simulink model "FINAL_SIMULATION"  (R2017a)
settings: Solver=FixedStepDiscrete  StartTime=0.0  StopTime=1  FixedStep=1e-6  RelTol=1e-3
libraries: powerlib x18, simulink x2, powerlib_meascontrol x2
settings Model: Creator=M. Mahinur Rahman  LastModifiedBy=Junaed

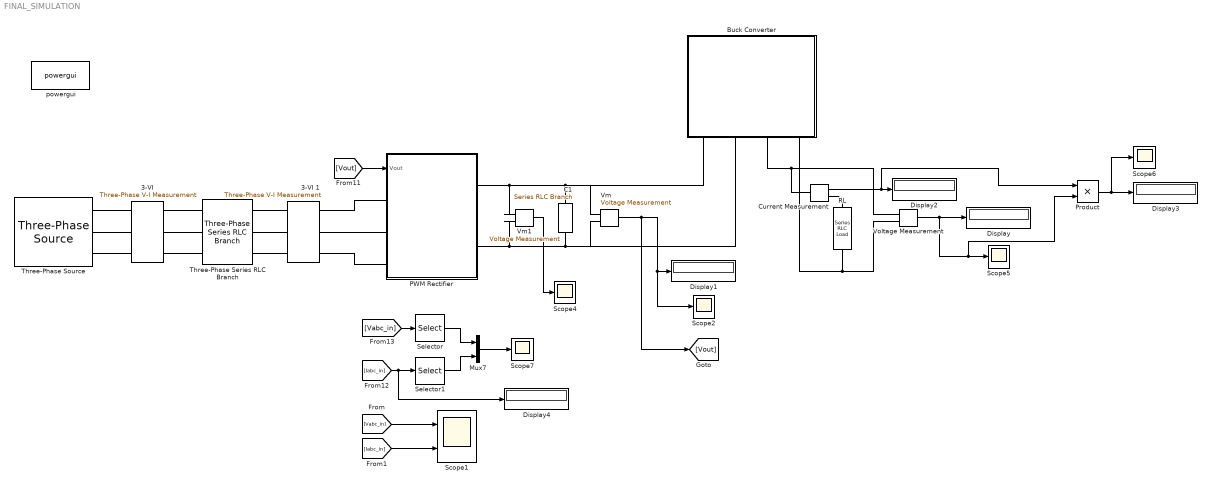
== system FINAL_SIMULATION ==
  " RL" : powerlib/Elements/Series RLC Load  LConnTagsString=a  RConnTagsString=__new0  NominalVoltage=87  NominalFrequency=50  ActivePower=2e3  InductivePower=0  CapacitivePower=0  Setx0=off  InitialVoltage=0  SetiL0=off  InitialCurrent=0  Measurements=None  LoadType=constant Z
  "3-VI " : powerlib/Measurements/Three-Phase V-I Measurement  VoltageMeasurement=phase-to-ground  SetLabelV=on  LabelV=Vabc_in  Vpu=off  VpuLL=off  CurrentMeasurement=yes  SetLabelI=on  LabelI=Iabc_in  Ipu=off  Pbase=100e6  Vbase=500e3  OutputType=Complex  PhasorSimulation=off  PSBequivalent=0
  3-VI 1 : powerlib/Measurements/Three-Phase V-I Measurement  VoltageMeasurement=phase-to-ground  SetLabelV=on  LabelV=Vabc_sw  Vpu=off  VpuLL=off  CurrentMeasurement=yes  SetLabelI=on  LabelI=Iabc_sw  Ipu=off  Pbase=100e6  Vbase=500e3  OutputType=Complex  PhasorSimulation=off  PSBequivalent=0
  Buck Converter : Subsystem
  C1 : powerlib/Elements/Series RLC Branch  LConnTagsString=__new0  RConnTagsString=__new0  BranchType=C  Resistance=1  Inductance=1e-3  SetiL0=off  InitialCurrent=0  Capacitance=1000e-6  Setx0=off  InitialVoltage=0  Measurements=None
  Current Measurement : powerlib/Measurements/Current Measurement  PhasorSimulation=off  OutputType=Complex  PSBequivalent=0
  Display{,1..4} (5 alike) : Display
  Mux7 : Mux  Inputs=2
  "PWM Rectifier " : Subsystem
  Product : Product
  Scope1 : Scope  NumInputPorts=2
  Scope{2,4..7} (5 alike) : Scope
  Selector : Selector  InputPortWidth=3  IndexOptions=Index vector (dialog)  Indices=[1]  OutputSizes=1
  Selector1 : Selector  InputPortWidth=3  IndexOptions=Index vector (dialog)  Indices=[1]  OutputSizes=1
  Three-Phase Series RLC Branch : powerlib/Elements/Three-Phase Series RLC Branch  LConnTagsString=A|B|C  RConnTagsString=A|B|C  BranchType=RL  Resistance=1  Inductance=5e-3  Capacitance=1e-6  Measurements=None
  Three-Phase Source : powerlib/Electrical Sources/Three-Phase Source  InternalConnection=Yg  VoltagePhases=off  Voltage=400  PhaseAngle=0  Voltage_phases=[25e3 25e3 25e3]/sqrt(3)  PhaseAngles_phases=[0 -120 +120]  Frequency=50  NonIdealSource=off  SpecifyImpedance=off  Resistance=0.8929  Inductance=16.58e-3  ShortCircuitLevel=100e6  BaseVoltage=25e3  XRratio=7  BusType=swing  Pref=10e3  Qref=0  Prefabc=[10e3, 10e3, 10e3]  Qrefabc=[0, 0, 0]  Qmin=-inf  Qmax=inf
  Vm : powerlib/Measurements/Voltage Measurement  PhasorSimulation=off  OutputType=Complex  PSBequivalent=0
  Vm1 : powerlib/Measurements/Voltage Measurement  PhasorSimulation=off  OutputType=Complex  PSBequivalent=0
  Voltage Measurement : powerlib/Measurements/Voltage Measurement  PhasorSimulation=off  OutputType=Complex  PSBequivalent=0
  powergui : powerlib/powergui  Priority=1  SimulationMode=Discrete  SampleTime=1e-6  frequency=60  Iterations=50  frequencyindice=50  Pbase=100e6  ErrMax=1e-4  UnitsV=kV  UnitsW=MW  buscounter=0  FunctionMessages=off  echomessages=off  EnableUseOfTLC=off  CurrentSourceSwitches=off  DisableSnubberDevices=off  DisableRonSwitches=off  DisableVfSwitches=off  DisplayEquations=off  SolverType=Tustin/Backward Euler (TBE)  Interpol=off  ExternalGateDelay=off  methode=off  Ts=100  x0status=blocks  SPID=off  SwTol=0  HookPort=off  RestoreLinks=warning  ResistiveCurrentMeasurement=off  Frange=[0:2:500]  Ylog=off  Xlog=on  ShowGrid=off  save=off  variable=ZData  structure=0  ZoomFFT=off  StartTime=0.0  cycles=1  DisplayStyle=1  fundamental=60  FreqAxis=off  MaxFrequency=1000  frequencyindicesteady=1  RmsSteady=1  display=off
  wires:
  [Iabc_in] -> Scope1/2
  [Vabc_in] -> Scope1/1
  Vm1/1 -> Scope4/1
  [Vabc_in] -> Selector/1
  [Iabc_in] -> Display4/1, Selector1/1
  Selector/1 -> Mux7/1
  Selector1/1 -> Mux7/2
  Mux7/1 -> Scope7/1
  Voltage Measurement/1 -> Display/1, Product/2, Scope5/1
  [Vout] -> "PWM Rectifier "/1(Vout)
  Vm/1 -> Scope2/1, Display1/1, [Vout]
  Current Measurement/1 -> Product/1, Display2/1
  Product/1 -> Scope6/1, Display3/1
  connections:
  C1/LConn1 -- Vm/LConn1 -- Buck Converter/LConn1 -- Vm1/LConn1 -- "PWM Rectifier "/RConn1
  C1/RConn1 -- Vm/LConn2 -- Buck Converter/LConn2 -- Vm1/LConn2 -- "PWM Rectifier "/RConn2
  "3-VI "/LConn1 -- Three-Phase Source/RConn1
  Three-Phase Source/RConn2 -- "3-VI "/LConn2
  Three-Phase Source/RConn3 -- "3-VI "/LConn3
  "3-VI "/RConn1 -- Three-Phase Series RLC Branch/LConn1
  "3-VI "/RConn2 -- Three-Phase Series RLC Branch/LConn2
  "3-VI "/RConn3 -- Three-Phase Series RLC Branch/LConn3
  3-VI 1/LConn3 -- Three-Phase Series RLC Branch/RConn3
  3-VI 1/LConn2 -- Three-Phase Series RLC Branch/RConn2
  3-VI 1/LConn1 -- Three-Phase Series RLC Branch/RConn1
  3-VI 1/RConn1 -- "PWM Rectifier "/LConn1
  3-VI 1/RConn2 -- "PWM Rectifier "/LConn2
  3-VI 1/RConn3 -- "PWM Rectifier "/LConn3
  Voltage Measurement/LConn1 -- Current Measurement/LConn1 -- Buck Converter/LConn3
  " RL"/RConn1 -- Voltage Measurement/LConn2 -- Buck Converter/LConn4
  Current Measurement/RConn1 -- " RL"/LConn1

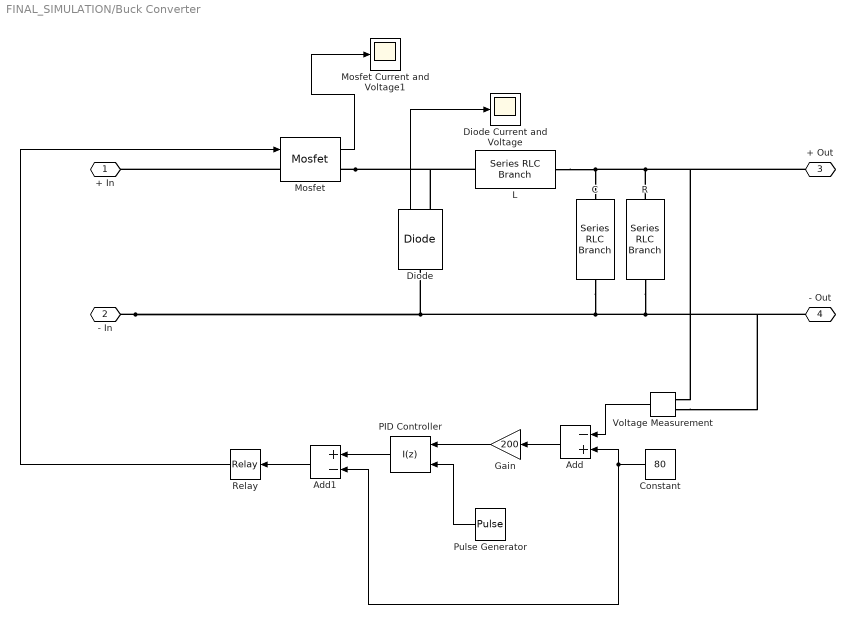
== system FINAL_SIMULATION/Buck Converter ==
  Add : Sum  Inputs=-+
  Add1 : Sum  Inputs=+-
  C : powerlib/Elements/Series RLC Branch  LConnTagsString=__new0  RConnTagsString=__new0  BranchType=C  Resistance=1  Inductance=1e-3  SetiL0=off  InitialCurrent=0  Capacitance=2.5e-5  Setx0=off  InitialVoltage=0  Measurements=None
  Constant : Constant  Value=80
  Diode : powerlib/Power Electronics/Diode  Ron=0.001  Lon=0  Vf=0.8  IC=0  UseSnubber=0  Rs=500  Cs=250e-9  Measurements=on
  Diode Current and Voltage : Scope
  Gain : Gain  Gain=200
  L : powerlib/Elements/Series RLC Branch  LConnTagsString=__new0  RConnTagsString=__new0  BranchType=L  Resistance=1  Inductance=0.34182  SetiL0=off  InitialCurrent=0  Capacitance=1e-6  Setx0=off  InitialVoltage=0  Measurements=None
  Mosfet : powerlib/Power Electronics/Mosfet  Ron=0.1  Lon=0  Rd=0.01  Vfd=0  IC=0  Rs=1e5  Cs=inf  Measurements=on
  Mosfet Current and Voltage1 : Scope
  PID Controller : simulink/Continuous/PID Controller  Controller=I  TimeDomain=Discrete-time  SampleTime=-1  IntegratorMethod=Forward Euler  FilterMethod=Forward Euler  Form=Parallel  UseFilter=on  ControllerParametersSource=internal  P=.001  I=40000  D=0  N=100  InitialConditionSource=internal  InitialConditionForIntegrator=0  InitialConditionForFilter=0  ExternalReset=falling  LimitOutput=off  UpperSaturationLimit=inf  LowerSaturationLimit=-inf  LinearizeAsGain=on  AntiWindupMode=none  Kb=1  TrackingMode=off  Kt=1  PParamMin=[]  PParamMax=[]  IParamMin=[]  IParamMax=[]  DParamMin=[]  DParamMax=[]  NParamMin=[]  NParamMax=[]  KbParamMin=[]  KbParamMax=[]  KtParamMin=[]  KtParamMax=[]  POutMin=[]  POutMax=[]  IOutMin=[]  IOutMax=[]  DOutMin=[]  DOutMax=[]  NOutMin=[]  NOutMax=[]  KbOutMin=[]  KbOutMax=[]  KtOutMin=[]  KtOutMax=[]  IntegratorOutMin=[]  IntegratorOutMax=[]  FilterOutMin=[]  FilterOutMax=[]  SumOutMin=[]  SumOutMax=[]  SumI1OutMin=[]  SumI1OutMax=[]  SumI2OutMin=[]  SumI2OutMax=[]  SumI3OutMin=[]  SumI3OutMax=[]  SumDOutMin=[]  SumDOutMax=[]  SaturationOutMin=[]  SaturationOutMax=[]  IntegratorContinuousStateAttributes=''  IntegratorStateMustResolveToSignalObject=off  IntegratorRTWStateStorageClass=Auto  FilterContinuousStateAttributes=''  FilterStateMustResolveToSignalObject=off  FilterRTWStateStorageClass=Auto  DifferentiatorICPrevScaledInput=0  DifferentiatorOutMin=[]  DifferentiatorOutMax=[]  InitialConditionSetting=State (most efficient)
  Pulse Generator : DiscretePulseGenerator  PulseType=Time based  Period=1/10000  PulseWidth=20
  R : powerlib/Elements/Series RLC Branch  LConnTagsString=__new0  RConnTagsString=__new0  BranchType=R  Resistance=20  Inductance=1e-3  SetiL0=off  InitialCurrent=0  Capacitance=1e-6  Setx0=off  InitialVoltage=0  Measurements=None
  Relay : Relay
  Voltage Measurement : powerlib/Measurements/Voltage Measurement  PhasorSimulation=off  OutputType=Complex  PSBequivalent=0
  + In : PMIOPort  Port=1  Side=Left
  - In : PMIOPort  Port=2  Side=Left
  + Out : PMIOPort  Port=3  Side=Left
  - Out : PMIOPort  Port=4  Side=Left
  wires:
  Diode/1 -> Diode Current and Voltage/1
  Mosfet/1 -> Mosfet Current and Voltage1/1
  Voltage Measurement/1 -> Add/1
  Constant/1 -> Add1/2, Add/2
  Add/1 -> Gain/1
  Gain/1 -> PID Controller/1
  Pulse Generator/1 -> PID Controller/2
  PID Controller/1 -> Add1/1
  Add1/1 -> Relay/1
  Relay/1 -> Mosfet/1
  connections:
  Mosfet/RConn1 -- Diode/RConn1 -- L/LConn1
  L/RConn1 -- Voltage Measurement/LConn1 -- + Out/RConn1 -- R/LConn1 -- C/LConn1
  - In/RConn1 -- Voltage Measurement/LConn2 -- - Out/RConn1 -- R/RConn1 -- C/RConn1 -- Diode/LConn1
  Mosfet/LConn1 -- + In/RConn1

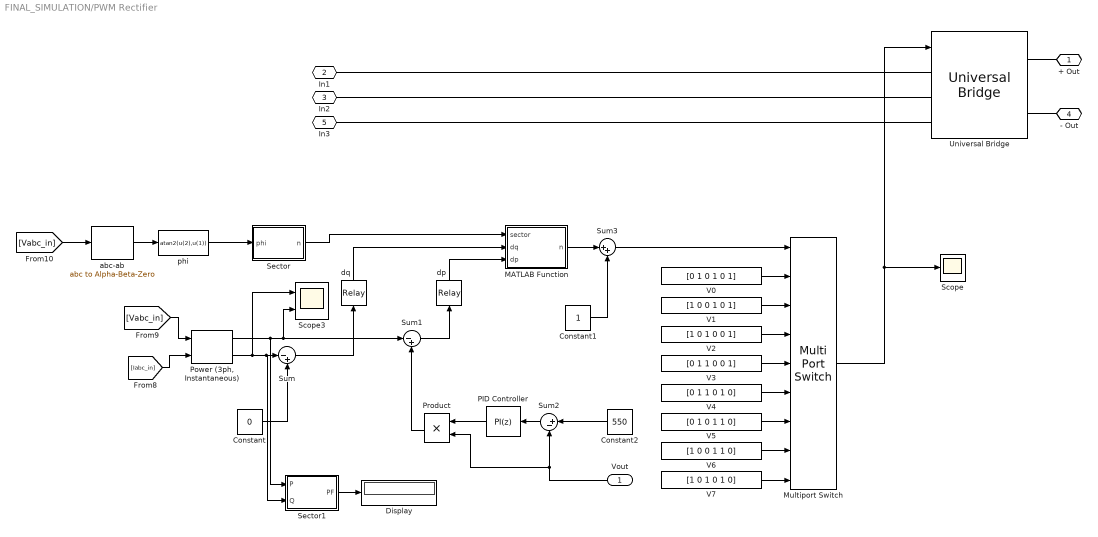
== system FINAL_SIMULATION/PWM Rectifier  ==
  Vout : Inport
  Constant : Constant  Value=0
  Constant1 : Constant
  Constant2 : Constant  Value=550
  Display : Display
  MATLAB Function : MATLAB Function  TreatAsAtomicUnit=on
  Multiport Switch : MultiPortSwitch  Inputs=8
  PID Controller : simulink/Continuous/PID Controller  Controller=PI  TimeDomain=Discrete-time  SampleTime=-1  IntegratorMethod=Forward Euler  FilterMethod=Forward Euler  Form=Parallel  UseFilter=on  ControllerParametersSource=internal  P=.001  I=.05  D=0  N=100  InitialConditionSource=internal  InitialConditionForIntegrator=0  InitialConditionForFilter=0  ExternalReset=none  LimitOutput=off  UpperSaturationLimit=inf  LowerSaturationLimit=-inf  LinearizeAsGain=on  AntiWindupMode=none  Kb=1  TrackingMode=off  Kt=1  PParamMin=[]  PParamMax=[]  IParamMin=[]  IParamMax=[]  DParamMin=[]  DParamMax=[]  NParamMin=[]  NParamMax=[]  KbParamMin=[]  KbParamMax=[]  KtParamMin=[]  KtParamMax=[]  POutMin=[]  POutMax=[]  IOutMin=[]  IOutMax=[]  DOutMin=[]  DOutMax=[]  NOutMin=[]  NOutMax=[]  KbOutMin=[]  KbOutMax=[]  KtOutMin=[]  KtOutMax=[]  IntegratorOutMin=[]  IntegratorOutMax=[]  FilterOutMin=[]  FilterOutMax=[]  SumOutMin=[]  SumOutMax=[]  SumI1OutMin=[]  SumI1OutMax=[]  SumI2OutMin=[]  SumI2OutMax=[]  SumI3OutMin=[]  SumI3OutMax=[]  SumDOutMin=[]  SumDOutMax=[]  SaturationOutMin=[]  SaturationOutMax=[]  IntegratorContinuousStateAttributes=''  IntegratorStateMustResolveToSignalObject=off  IntegratorRTWStateStorageClass=Auto  FilterContinuousStateAttributes=''  FilterStateMustResolveToSignalObject=off  FilterRTWStateStorageClass=Auto  DifferentiatorICPrevScaledInput=0  DifferentiatorOutMin=[]  DifferentiatorOutMax=[]  InitialConditionSetting=State (most efficient)
  "Power (3ph, Instantaneous)" : powerlib_meascontrol/Measurements/Power (3ph, Instantaneous)
      settings: SourceProductName=Simscape Power Systems
  Product : Product
  Scope : Scope
  Scope3 : Scope  NumInputPorts=2
  Sector : MATLAB Function  TreatAsAtomicUnit=on
  Sector1 : MATLAB Function  TreatAsAtomicUnit=on
  Sum : Sum  Inputs=|-+
  Sum1 : Sum  Inputs=|-+
  Sum2 : Sum  Inputs=|+-
  Sum3 : Sum  Inputs=|++
  Universal Bridge : powerlib/Power Electronics/Universal Bridge  Arms=3  SnubberResistance=1e5  SnubberCapacitance=inf  Device=MOSFET / Diodes  Ron=1e-3  Lon=0  ForwardVoltages="[  0  0  ]"  ForwardVoltage=0  GTOparameters=[ 10e-6 , 20e-6 ]  IGBTparameters=[ 1e-6 , 2e-6 ]  Measurements=All voltages and currents  Measurements_2=None  converterType=Rectifier
  V0 : Constant  Value=[0 1 0 1 0 1]
  V1 : Constant  Value=[1 0 0 1 0 1]
  V2 : Constant  Value=[1 0 1 0 0 1]
  V3 : Constant  Value=[0 1 1 0 0 1]
  V4 : Constant  Value=[0 1 1 0 1 0]
  V5 : Constant  Value=[0 1 0 1 1 0]
  V6 : Constant  Value=[1 0 0 1 1 0]
  V7 : Constant  Value=[1 0 1 0 1 0]
  abc-ab : powerlib_meascontrol/Transformations/abc to Alpha-Beta-Zero
      settings: SourceProductName=Simscape Power Systems
  dp : Relay  OnSwitchValue=1  OffSwitchValue=-1
  dq : Relay  OnSwitchValue=1  OffSwitchValue=-1
  phi : Fcn  Expr=atan2(u(2),u(1))
  + Out : PMIOPort  Port=1  Side=Right
  In1 : PMIOPort  Port=2  Side=Left
  In2 : PMIOPort  Port=3  Side=Left
  - Out : PMIOPort  Port=4  Side=Right
  In3 : PMIOPort  Port=5  Side=Left
  wires:
  Constant/1 -> Sum/2
  Sum3/1 -> Multiport Switch/1
  Sum/1 -> dq/1
  V6/1 -> Multiport Switch/8
  Vout/1 -> Sum2/2, Product/2
  Sector/1(n) -> MATLAB Function/1(sector)
  V4/1 -> Multiport Switch/6
  V2/1 -> Multiport Switch/4
  Constant2/1 -> Sum2/1
  V3/1 -> Multiport Switch/5
  V1/1 -> Multiport Switch/3
  V5/1 -> Multiport Switch/7
  Constant1/1 -> Sum3/2
  dp/1 -> MATLAB Function/3(dp)
  "Power (3ph, Instantaneous)"/2 -> Scope3/1, Sector1/2(Q), Sum/1
  dq/1 -> MATLAB Function/2(dq)
  PID Controller/1 -> Product/1
  MATLAB Function/1(n) -> Sum3/1
  Sum1/1 -> dp/1
  [Iabc_in] -> "Power (3ph, Instantaneous)"/2
  Sum2/1 -> PID Controller/1
  V7/1 -> Multiport Switch/9
  [Vabc_in] -> abc-ab/1
  abc-ab/1 -> phi/1
  [Vabc_in] -> "Power (3ph, Instantaneous)"/1
  "Power (3ph, Instantaneous)"/1 -> Sector1/1(P), Scope3/2, Sum1/1
  Product/1 -> Sum1/2
  phi/1 -> Sector/1(phi)
  V0/1 -> Multiport Switch/2
  Sector1/1(PF) -> Display/1
  Multiport Switch/1 -> Scope/1, Universal Bridge/1
  connections:
  In3/RConn1 -- Universal Bridge/LConn3
  In1/RConn1 -- Universal Bridge/LConn1
  + Out/RConn1 -- Universal Bridge/RConn1
  In2/RConn1 -- Universal Bridge/LConn2
  - Out/RConn1 -- Universal Bridge/RConn2

== matlab function FINAL_SIMULATION/PWM Rectifier /MATLAB Function ==
  data: sector input; dq input; dp input; n output
function n = fcn(sector,dq,dp)
n = 0;
%sector 1
if(sector == 2) & (dp == 1) & (dq == 0)
    n = 1;
end
if(sector == 2) & (dp == 1) & (dq == 1)
    n = 0;
end
if(sector == 2) & (dp == 0) & (dq == 0)
    n = 1;
end
if(sector == 2) & (dp == 0) & (dq == 1)
    n = 2;
end

if(sector == 3) & (dp == 1) & (dq == 0)
    n = 7;
end
if(sector == 3) & (dp == 1) & (dq == 1)
    n = 7;
end
if(sector == 3) & (dp == 0) & (dq == 0)
    n = 1;
end
if(sector == 3) & (dp == 0) & (dq == 1)
    n = 2;
end

%SECTOR 2
if(sector == 4) & (dp == 1) & (dq == 0)
    n = 2;
end
if(sector == 4) & (dp == 1) & (dq == 1)
    n = 0;
end
if(sector == 4) & (dp == 0) & (dq == 0)
    n = 2;
end
if(sector == 4) & (dp == 0) & (dq == 1)
    n = 3;
end

if(sector == 5) & (dp == 1) & (dq == 0)
    n = 7;
end
if(sector == 5) & (dp == 1) & (dq == 1)
    n = 7;
end
if(sector == 5) & (dp == 0) & (dq == 0)
    n = 2;
end
if(sector == 5) & (dp == 0) & (dq == 1)
    n = 3;
end

%Sector 3 

if(sector == 6) & (dp == 1) & (dq == 0)
    n = 3;
end
if(sector == 6) & (dp == 1) & (dq == 1)
    n = 0;
end
if(sector == 6) & (dp == 0) & (dq == 0)
    n = 3;
end
if(sector == 6) & (dp == 0) & (dq == 1)
    n = 4;
end

if(sector == 7) & (dp == 1) & (dq == 0)
    n = 7;
end
if(sector == 7) & (dp == 1) & (dq == 1)
    n = 7;
end
if(sector == 7) & (dp == 0) & (dq == 0)
    n = 3;
end
if(sector == 7) & (dp == 0) & (dq == 1)
    n = 4;
end

%Sector 4
if(sector == 8) & (dp == 1) & (dq == 0)
    n = 4;
end
if(sector == 8) & (dp == 1) & (dq == 1)
    n = 0;
end
if(sector == 8) & (dp == 0) & (dq == 0)
    n = 4;
end
if(sector == 8) & (dp == 0) & (dq == 1)
    n = 5;
end

if(sector == 9) & (dp == 1) & (dq == 0)
    n = 7;
end
if(sector == 9) & (dp == 1) & (dq == 1)
    n = 7;
end
if(sector == 9) & (dp == 0) & (dq == 0)
    n = 4;
end
if(sector == 9) & (dp == 0) & (dq == 1)
    n = 5;
end

%Sector 5
if(sector == 10) & (dp == 1) & (dq == 0)
    n = 5;
end
if(sector == 10) & (dp == 1) & (dq == 1)
    n = 0;
end
if(sector == 10) & (dp == 0) & (dq == 0)
    n = 5;
end
if(sector == 10) & (dp == 0) & (dq == 1)
    n = 6;
end

if(sector == 11) & (dp == 1) & (dq == 0)
    n = 7;
end
if(sector == 11) & (dp == 1) & (dq == 1)
    n = 7;
end
if(sector == 11) & (dp == 0) & (dq == 0)
    n = 5;
end
if(sector == 11) & (dp == 0) & (dq == 1)
    n = 6;
end
%Sector 6
if(sector == 12) & (dp == 1) & (dq == 0)
    n = 6;
end
if(sector == 12) & (dp == 1) & (dq == 1)
    n = 0;
end
if(sector == 12) & (dp == 0) & (dq == 0)
    n = 6;
end
if(sector == 12) & (dp == 0) & (dq == 1)
    n = 1;
end

if(sector == 1) & (dp == 1) & (dq == 0)
    n = 7;
end
if(sector == 1) & (dp == 1) & (dq == 1)
    n = 7;
end
if(sector == 1) & (dp == 0) & (dq == 0)
    n = 6;
end
if(sector == 1) & (dp == 0) & (dq == 1)
    n = 1;
end

== matlab function FINAL_SIMULATION/PWM Rectifier /Sector ==
  data: phi input; n output
function n = fcn(phi)

n = 0;

if(phi >= 0) & (phi < pi/6)
    n = 2;
end

if(phi >= pi/6) & (phi < pi/3)
    n = 3;
end

if(phi >= pi/3) & (phi < pi/2)
    n = 4;
end

if(phi >= pi/2) & (phi < 2*pi/3)
    n = 5;
end

if(phi >= 2*pi/3) & (phi < 5*pi/6)
    n = 6;
end

if(phi >= 5*pi/6) & (phi < pi)
    n = 7;
end

if(phi >= -pi) & (phi < -5*pi/6)
    n = 8;
end

if(phi >= -5*pi/6) & (phi < -2*pi/3)
    n = 9;
end

if(phi >= -2*pi/3) & (phi < -pi/2)
    n = 10;
end

if(phi >= -pi/2) & (phi < -pi/3)
    n = 11;
end

if(phi >= -pi/3) & (phi < -pi/6)
    n = 12;
end

if(phi >= -pi/6) & (phi < 0)
    n = 1;
end

== matlab function FINAL_SIMULATION/PWM Rectifier /Sector1 ==
  data: P input; PF output; Q input
function PF = fcn(P,Q)
PF = P / sqrt(P^2 + Q^2) ;

end
